simulink model "Single_Phase_without_DC_machine"  (R2022a)
settings: Solver=VariableStepAuto  StartTime=0.0  StopTime=2  MaxStep=1/(50*100)  RelTol=1e-3
libraries: spsDiodeLib x4, spsVoltageMeasurementLib x2, spsMeanLib x2, spsRMSLib x2, spsACVoltageSourceLib x1, spspowerguiLib x1
settings Model: Creator=mohit  LastModifiedBy=mohit
settings DataIOCC: ReturnWorkspaceOutputs=off

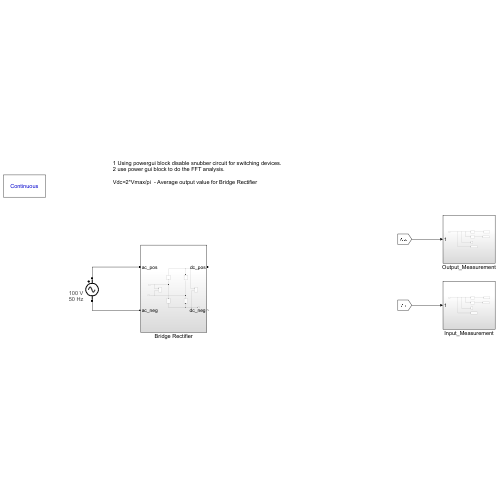
[thumbnail: Simulink's stored preview of the top-level diagram]
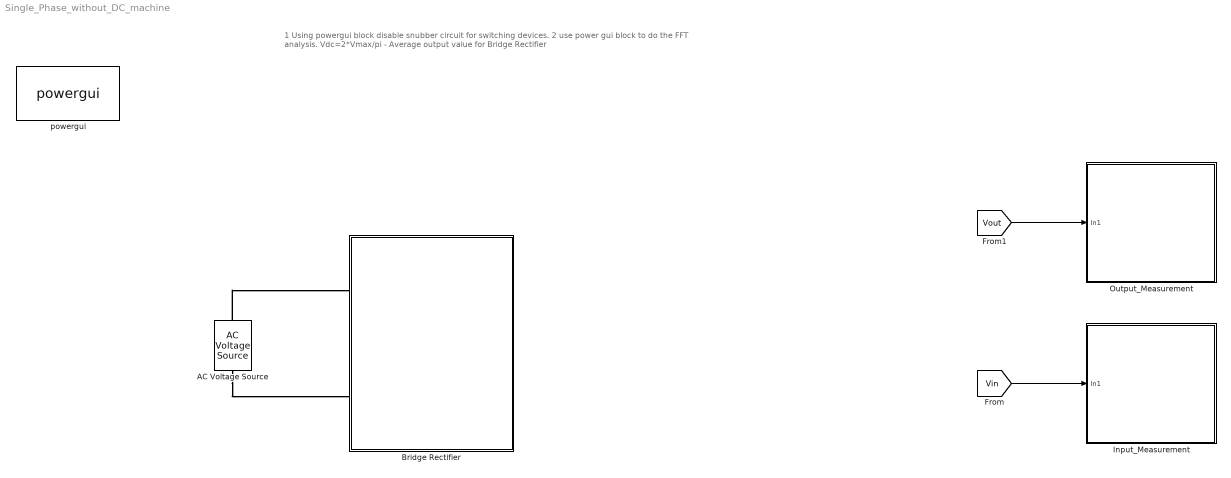
== system Single_Phase_without_DC_machine ==
  note: 1 Using powergui block disable snubber circuit for switching devices.
      | 2 use power gui block to do the FFT analysis.
      |
      | Vdc=2*Vmax/pi - Average output value for Bridge Rectifier
  AC Voltage Source : spsACVoltageSourceLib/AC Voltage Source  Amplitude=100  Phase=0  Frequency=50  SampleTime=0  Measurements=None  BusType=swing  Pref=10e3  Qref=0  Qmin=-inf  Qmax=+inf
      settings: AttributesFormatString=|
      | %<Amplitude> V
      | %<Frequency> Hz
  Bridge Rectifier : Subsystem
  Input_Measurement : Subsystem
  Output_Measurement : Subsystem
  powergui : spspowerguiLib/powergui  Priority=1  SimulationMode=Continuous  SampleTime=50e-6  frequency=60  Iterations=50  frequencyindice=50  Pbase=100e6  ErrMax=1e-4  UnitsV=kV  UnitsW=MW  buscounter=0  FunctionMessages=off  echomessages=off  EnableUseOfTLC=off  CurrentSourceSwitches=off  DisableSnubberDevices=on  DisableRonSwitches=off  DisableVfSwitches=off  DisplayEquations=on  AutomaticDiscreteSolvers=off  SolverType=Tustin/Backward Euler (TBE)  Interpol=off  ExternalGateDelay=off  methode=off  Ts=100  x0status=blocks  SPID=on  SwTol=0  HookPort=off  NonlinearTolerance=1e-4  nMaxIteration=100  ContinueOnMaxIteration=off  RestoreLinks=warning  ResistiveCurrentMeasurement=off  Frange=[0:2:500]  Ylog=off  Xlog=on  ShowGrid=off  save=off  variable=ZData  structure=0  ZoomFFT=off  StartTime=0.0  cycles=1  DisplayStyle=1  fundamental=60  FreqAxis=off  MaxFrequency=1000  frequencyindicesteady=1  RmsSteady=1  display=off
  wires:
  [Vin] -> Input_Measurement/1(In1)
  [Vout] -> Output_Measurement/1(In1)
  connections:
  AC Voltage Source/RConn1 -- Bridge Rectifier/LConn1
  AC Voltage Source/LConn1 -- Bridge Rectifier/LConn2

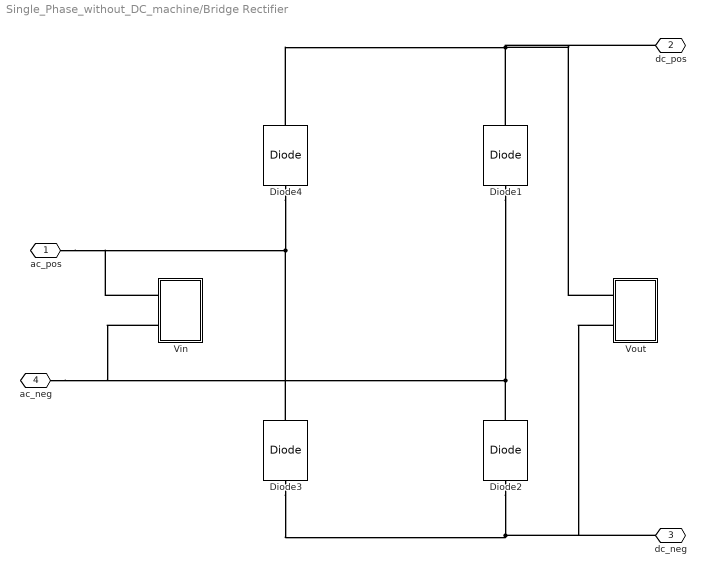
== system Single_Phase_without_DC_machine/Bridge Rectifier ==
  Diode{1..4} (4 alike) : spsDiodeLib/Diode  Ron=0.001  Lon=0  Vf=0.8  IC=0  UseSnubber=0  Rs=500  Cs=250e-9  Measurements=off
  Vin : Subsystem
  Vout : Subsystem
  ac_pos : PMIOPort  Side=Left
  dc_pos : PMIOPort  Port=2  Side=Right
  dc_neg : PMIOPort  Port=3  Side=Right
  ac_neg : PMIOPort  Port=4  Side=Left
  connections:
  Diode4/RConn1 -- Vout/LConn1 -- dc_pos/RConn1 -- Diode1/RConn1
  Diode3/RConn1 -- Vin/LConn1 -- ac_pos/RConn1 -- Diode4/LConn1
  Diode2/LConn1 -- Vout/LConn2 -- dc_neg/RConn1 -- Diode3/LConn1
  Diode1/LConn1 -- Vin/LConn2 -- ac_neg/RConn1 -- Diode2/RConn1

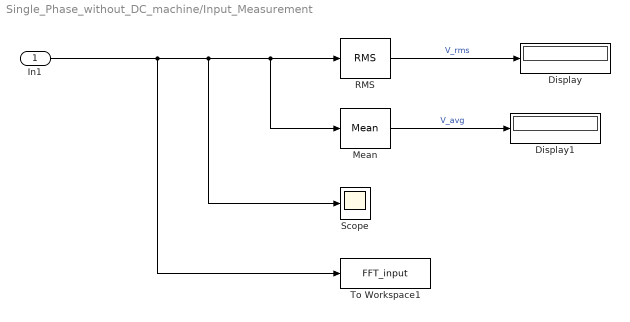
== system Single_Phase_without_DC_machine/Input_Measurement ==
  In1 : Inport
  Display : Display
  Display1 : Display
  Mean : spsMeanLib/Mean  Freq=100  Vinit=0  Ts=0
  RMS : spsRMSLib/RMS  TrueRMS=on  Freq=100  RMSInit=0  Ts=0
  Scope : Scope
  To Workspace1 : ToWorkspace  VariableName=FFT_input  SaveFormat=Structure With Time  SampleTime=-1
  wires:
  Mean/1 -> Display1/1  "V_avg"
  RMS/1 -> Display/1  "V_rms"
  In1/1 -> To Workspace1/1, Scope/1, Mean/1, RMS/1

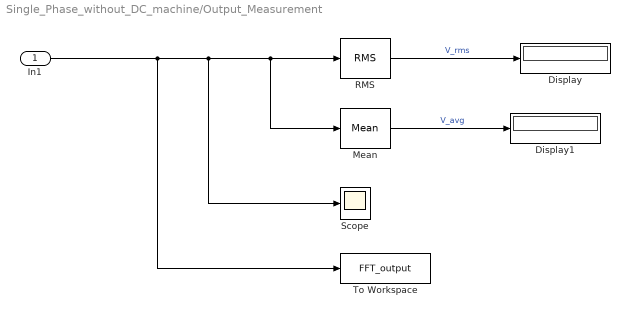
== system Single_Phase_without_DC_machine/Output_Measurement ==
  In1 : Inport
  Display : Display
  Display1 : Display
  Mean : spsMeanLib/Mean  Freq=100  Vinit=0  Ts=0
  RMS : spsRMSLib/RMS  TrueRMS=on  Freq=100  RMSInit=0  Ts=0
  Scope : Scope
  To Workspace : ToWorkspace  VariableName=FFT_output  SaveFormat=Structure With Time  SampleTime=-1
  wires:
  Mean/1 -> Display1/1  "V_avg"
  RMS/1 -> Display/1  "V_rms"
  In1/1 -> To Workspace/1, Scope/1, Mean/1, RMS/1

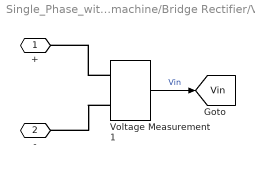
== system Single_Phase_without_DC_machine/Bridge Rectifier/Vin ==
  Voltage Measurement1 : spsVoltageMeasurementLib/Voltage Measurement  PhasorSimulation=off  OutputType=Complex  PSBequivalent=0
  + : PMIOPort  Side=Left
  - : PMIOPort  Port=2  Side=Left
  tag scope: Vin=global
  wires:
  Voltage Measurement1/1 -> [Vin]  "Vin"
  connections:
  Voltage Measurement1/LConn1 -- +/RConn1
  Voltage Measurement1/LConn2 -- -/RConn1

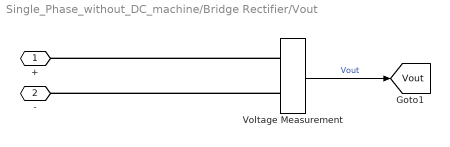
== system Single_Phase_without_DC_machine/Bridge Rectifier/Vout ==
  Voltage Measurement : spsVoltageMeasurementLib/Voltage Measurement  PhasorSimulation=off  OutputType=Complex  PSBequivalent=0
  + : PMIOPort  Side=Left
  - : PMIOPort  Port=2  Side=Left
  tag scope: Vout=global
  wires:
  Voltage Measurement/1 -> [Vout]  "Vout"
  connections:
  Voltage Measurement/LConn2 -- -/RConn1
  Voltage Measurement/LConn1 -- +/RConn1
